simulink model "MRAC_Indireto_Caso_Escalar_07_03_2018"  (R2013b)
settings: Solver=ode45  StartTime=0.0  StopTime=50  RelTol=1e-3
libraries: simulink x1
settings Model: Creator=Eduardo  LastModifiedBy=Eduardo

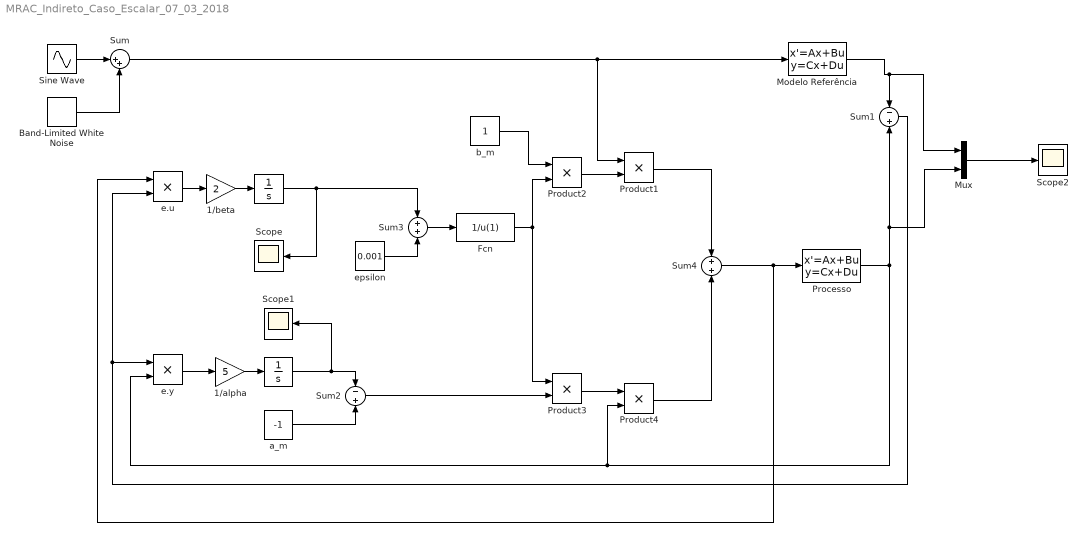
== system MRAC_Indireto_Caso_Escalar_07_03_2018 ==
  " " : Integrator
  "   " : Integrator
  1/alpha : Gain  Gain=5
  1/beta : Gain  Gain=2
  Band-Limited White Noise : simulink/Sources/Band-Limited White Noise  Cov=[0.1]  Ts=0.1  seed=[23341]
  Fcn : Fcn  Expr=1/u(1)
  Modelo Referência : StateSpace  A=-1  D=0  X0=0
  Mux : Mux  Inputs=2
  Processo : StateSpace  A=-2  D=0  X0=0
  Product{1..4} (4 alike) : Product
  Scope : Scope
  Scope1 : Scope
  Scope2 : Scope
      settings: SaveName=ScopeData2
  Sine Wave : Sin  SampleTime=0
  Sum : Sum  Inputs=|++
  Sum1 : Sum  Inputs=-|+
  Sum2 : Sum  Inputs=-|+
  Sum3 : Sum  Inputs=+|+
  Sum4 : Sum  Inputs=+|+
  a_m : Constant  Value=-1
  b_m : Constant
  e.u : Product
  e.y : Product
  "epsilon " : Constant  Value=0.001
  wires:
  Sine Wave/1 -> Sum/1
  Band-Limited White Noise/1 -> Sum/2
  Sum/1 -> Product1/1, Modelo Referência/1
  Modelo Referência/1 -> Mux/1, Sum1/1
  Processo/1 -> Mux/2, Sum1/2, Product4/2, e.y/2
  Sum1/1 -> e.u/2, e.y/1
  e.y/1 -> 1/alpha/1
  e.u/1 -> 1/beta/1
  1/beta/1 -> "   "/1
  1/alpha/1 -> " "/1
  " "/1 -> Scope1/1, Sum2/1
  a_m/1 -> Sum2/2
  "   "/1 -> Sum3/1, Scope/1
  Sum4/1 -> e.u/1, Processo/1
  "epsilon "/1 -> Sum3/2
  Sum3/1 -> Fcn/1
  b_m/1 -> Product2/1
  Fcn/1 -> Product2/2, Product3/1
  Product2/1 -> Product1/2
  Sum2/1 -> Product3/2
  Product3/1 -> Product4/1
  Product4/1 -> Sum4/2
  Product1/1 -> Sum4/1
  Mux/1 -> Scope2/1
